simulink model "deadtime_compensation"  (R2020a)
settings: Solver=ode45  StartTime=0.0  StopTime=0.15  FixedStep=0.0000001  RelTol=1e-3
libraries: powerlib_meascontrol x13, powerlib x8, simulink x2, mcbcontrolslib x1
settings Model: Creator=ZJX  LastModifiedBy=ZJX
settings DebuggingCC: UnconnectedInputMsg=none  UnconnectedOutputMsg=none  UnconnectedLineMsg=none
settings ModelReferenceCC: EnableRefExpFcnMdlSchedulingChecks=off
settings RTWCC: Description=Generic Real-Time Target

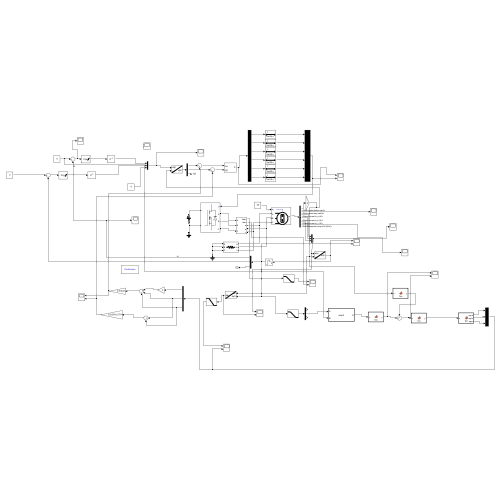
[thumbnail: Simulink's stored preview of the top-level diagram]
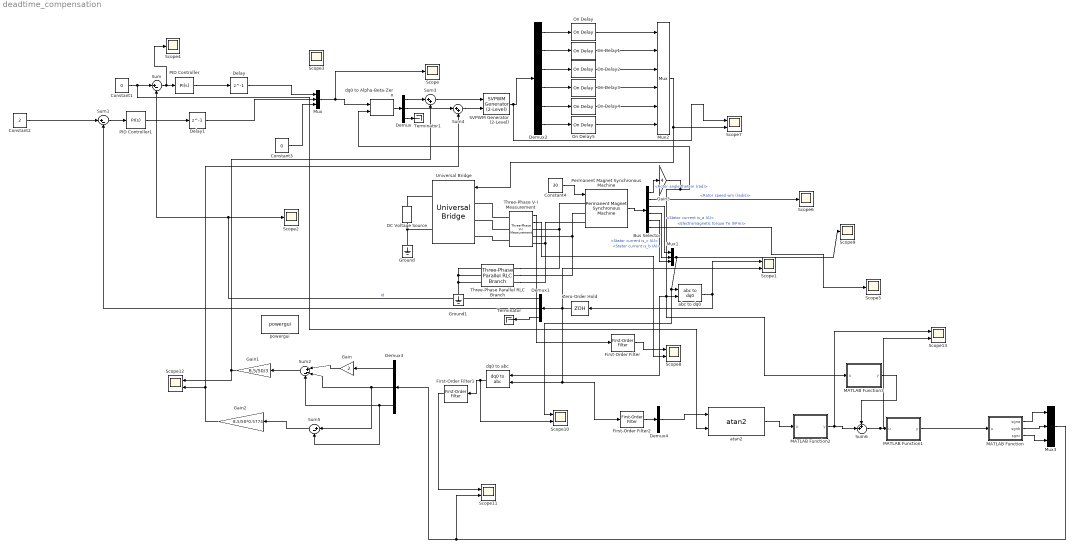
== system deadtime_compensation ==
  Bus Selector : BusSelector  OutputSignals=Rotor angle thetam (rad),Rotor speed wm (rad/s),Stator current is_a (A),Stator current is_b (A),Stator current is_c (A),Electromagnetic torque Te (N*m)
  Constant1 : Constant  Value=0
  Constant2 : Constant  Value=2
  Constant3 : Constant  Value=0
  Constant4 : Constant  Value=30
  DC Voltage Source : powerlib/Electrical Sources/DC Voltage Source  Amplitude=24  Measurements=None
  Delay : Delay  DelayLength=1  InitialCondition=0  SampleTime=0.00005
  Delay1 : Delay  DelayLength=1  InitialCondition=0  SampleTime=0.00005
  Demux{,1,3..4} (4 alike) : Demux  Outputs=3
  Demux2 : Demux  Outputs=6
  First-Order Filter : powerlib_meascontrol/Filters/First-Order Filter  FilterType=Lowpass  Tc=10e-4  Ts=0  Initialize=on  Vac_Init=[0, 0, 60]  Vdc_Init=0  PlotResponse=off  FreqRange="[0,  200,  1]"
  First-Order Filter1 : powerlib_meascontrol/Filters/First-Order Filter  FilterType=Lowpass  Tc=10e-5  Ts=0  Initialize=on  Vac_Init=[0, 0, 60]  Vdc_Init=0  PlotResponse=off  FreqRange="[0,  200,  1]"
  First-Order Filter2 : powerlib_meascontrol/Filters/First-Order Filter  FilterType=Lowpass  Tc=10e-6  Ts=0  Initialize=on  Vac_Init=[0, 0, 60]  Vdc_Init=0  PlotResponse=off  FreqRange="[0,  200,  1]"
  Gain : Gain  Gain=2
  Gain1 : Gain  Gain=8.5/50/3
  Gain2 : Gain  Gain=8.5/50*0.5774
  Gain3 : Gain  Gain=4
  Ground : powerlib/Elements/Ground  LConnTagsString=a
  Ground1 : powerlib/Elements/Ground  LConnTagsString=a
  MATLAB Function : MATLAB Function  TreatAsAtomicUnit=on
  MATLAB Function1 : MATLAB Function  TreatAsAtomicUnit=on
  MATLAB Function2 : MATLAB Function  TreatAsAtomicUnit=on
  MATLAB Function3 : MATLAB Function  TreatAsAtomicUnit=on
  Mux : Mux  Inputs=3
  Mux1 : Mux  Inputs=3
  Mux2 : Mux  Inputs=6
  Mux3 : Mux  Inputs=3
  On Delay{,1..5} (6 alike) : powerlib_meascontrol/Logic/On Delay  DelayType=On delay  delay=0.000005  ic=0  Ts=0
  PID Controller : simulink/Continuous/PID Controller  Controller=PI  Form=Parallel  TimeDomain=Continuous-time  UseExternalTs=off  SampleTime=-1  IntegratorMethod=Forward Euler  ControllerParametersSource=internal  P=0.00017*200  I=0.00017*200* 0.1 / 0.00017  D=0  N=100  UseFilter=on  TunerSelectOption=Frequency Response Based  ZeroCross=off  InitialConditionSource=internal  InitialConditionForIntegrator=0  InitialConditionForFilter=0  DifferentiatorICPrevScaledInput=0  ExternalReset=none  TrackingMode=off  Kt=1  LimitOutput=on  UpperSaturationLimit=1  LowerSaturationLimit=-1  LinearizeAsGain=off  AntiWindupMode=clamping  Kb=1  POutMin=[]  POutMax=[]  IOutMin=[]  IOutMax=[]  DOutMin=[]  DOutMax=[]  NOutMin=[]  NOutMax=[]  SumOutMin=[]  SumOutMax=[]  SaturationOutMin=[]  SaturationOutMax=[]  PParamMin=[]  PParamMax=[]  IParamMin=[]  IParamMax=[]  DParamMin=[]  DParamMax=[]  NParamMin=[]  NParamMax=[]  KbParamMin=[]  KbParamMax=[]  KtParamMin=[]  KtParamMax=[]  KbOutMin=[]  KbOutMax=[]  KtOutMin=[]  KtOutMax=[]  IntegratorOutMin=[]  IntegratorOutMax=[]  FilterOutMin=[]  FilterOutMax=[]  SumI1OutMin=[]  SumI1OutMax=[]  SumI2OutMin=[]  SumI2OutMax=[]  SumI3OutMin=[]  SumI3OutMax=[]  SumI4OutMin=[]  SumI4OutMax=[]  SumDOutMin=[]  SumDOutMax=[]  DifferentiatorOutMin=[]  DifferentiatorOutMax=[]  FilterDiffOutCoefMin=[]  FilterDiffOutCoefMax=[]  ReciprocalOutMin=[]  ReciprocalOutMax=[]  SumDenOutMin=[]  SumDenOutMax=[]  SumNumOutMin=[]  SumNumOutMax=[]  DivideOutMin=[]  DivideOutMax=[]  UdiffTsProdOutMin=[]  UdiffTsProdOutMax=[]  NTsProdOutMin=[]  NTsProdOutMax=[]  UintegralTsProdOutMin=[]  UintegralTsProdOutMax=[]  UngainTsProdOutMin=[]  UngainTsProdOutMax=[]  IntegratorContinuousStateAttributes=''  IntegratorStateMustResolveToSignalObject=off  IntegratorRTWStateStorageClass=Auto  FilterContinuousStateAttributes=''  FilterStateMustResolveToSignalObject=off  FilterRTWStateStorageClass=Auto  ParallelPVariant=InternalParameters  IdealPVariant=Disabled  IVariant=InternalParameters  DVariant=Disabled  IntegratorVariant=Continuous  SatVariant=Enabled  AWVariant=ContClampingParallel  PCopyVariant=Disabled  TRVariant=Disabled  FdbkBlocksVariant=Forward  IdealPFdbkVariant=Disabled  SatFdbkVariant=Disabled  DerivativeFilterVariant=Disabled  NVariant=Disabled  NCopyVariant=Disabled_SignalSpec  FilterICVariant=Disabled  IntegratorICVariant=InternalICs  ExternalResetVariant=Disabled  TRSumVariant=Passthrough  SumFdbkVariant=Disabled  SumVariant=Sum_PI  TsampFilterVariant=InternalTs  TsampNgainVariant=Passthrough  TsampIntegralVariant=Disabled_SignalSpec
  PID Controller1 : simulink/Continuous/PID Controller  Controller=PI  Form=Parallel  TimeDomain=Continuous-time  UseExternalTs=off  SampleTime=-1  IntegratorMethod=Forward Euler  ControllerParametersSource=internal  P=0.00017*200  I=0.00017*200* 0.1 / 0.00017  D=0  N=100  UseFilter=on  TunerSelectOption=Frequency Response Based  ZeroCross=off  InitialConditionSource=internal  InitialConditionForIntegrator=0  InitialConditionForFilter=0  DifferentiatorICPrevScaledInput=0  ExternalReset=none  TrackingMode=off  Kt=1  LimitOutput=on  UpperSaturationLimit=1  LowerSaturationLimit=-1  LinearizeAsGain=off  AntiWindupMode=clamping  Kb=1  POutMin=[]  POutMax=[]  IOutMin=[]  IOutMax=[]  DOutMin=[]  DOutMax=[]  NOutMin=[]  NOutMax=[]  SumOutMin=[]  SumOutMax=[]  SaturationOutMin=[]  SaturationOutMax=[]  PParamMin=[]  PParamMax=[]  IParamMin=[]  IParamMax=[]  DParamMin=[]  DParamMax=[]  NParamMin=[]  NParamMax=[]  KbParamMin=[]  KbParamMax=[]  KtParamMin=[]  KtParamMax=[]  KbOutMin=[]  KbOutMax=[]  KtOutMin=[]  KtOutMax=[]  IntegratorOutMin=[]  IntegratorOutMax=[]  FilterOutMin=[]  FilterOutMax=[]  SumI1OutMin=[]  SumI1OutMax=[]  SumI2OutMin=[]  SumI2OutMax=[]  SumI3OutMin=[]  SumI3OutMax=[]  SumI4OutMin=[]  SumI4OutMax=[]  SumDOutMin=[]  SumDOutMax=[]  DifferentiatorOutMin=[]  DifferentiatorOutMax=[]  FilterDiffOutCoefMin=[]  FilterDiffOutCoefMax=[]  ReciprocalOutMin=[]  ReciprocalOutMax=[]  SumDenOutMin=[]  SumDenOutMax=[]  SumNumOutMin=[]  SumNumOutMax=[]  DivideOutMin=[]  DivideOutMax=[]  UdiffTsProdOutMin=[]  UdiffTsProdOutMax=[]  NTsProdOutMin=[]  NTsProdOutMax=[]  UintegralTsProdOutMin=[]  UintegralTsProdOutMax=[]  UngainTsProdOutMin=[]  UngainTsProdOutMax=[]  IntegratorContinuousStateAttributes=''  IntegratorStateMustResolveToSignalObject=off  IntegratorRTWStateStorageClass=Auto  FilterContinuousStateAttributes=''  FilterStateMustResolveToSignalObject=off  FilterRTWStateStorageClass=Auto  ParallelPVariant=InternalParameters  IdealPVariant=Disabled  IVariant=InternalParameters  DVariant=Disabled  IntegratorVariant=Continuous  SatVariant=Enabled  AWVariant=ContClampingParallel  PCopyVariant=Disabled  TRVariant=Disabled  FdbkBlocksVariant=Forward  IdealPFdbkVariant=Disabled  SatFdbkVariant=Disabled  DerivativeFilterVariant=Disabled  NVariant=Disabled  NCopyVariant=Disabled_SignalSpec  FilterICVariant=Disabled  IntegratorICVariant=InternalICs  ExternalResetVariant=Disabled  TRSumVariant=Passthrough  SumFdbkVariant=Disabled  SumVariant=Sum_PI  TsampFilterVariant=InternalTs  TsampNgainVariant=Passthrough  TsampIntegralVariant=Disabled_SignalSpec
  Permanent Magnet Synchronous Machine : powerlib/Machines/Permanent Magnet Synchronous Machine  NbPhases=3  FluxDistribution=Sinusoidal  RotorType=Round  MechanicalLoad=Speed w  PresetModel=No  ShowDetailedParameters=on  MeasurementBus=off  Resistance=0.1  Inductance=8.5e-3  dqInductances=[8.5e-3,8.5e-3]  La=0.00017  MachineConstant=Torque Constant (N.m / A_peak)  Flux=0.016667  VoltageCst=12.092  TorqueCst=0.1  Flat=120  Mechanical=[0.00027 0.0004924 1 0]  PolePairs=4  InitialConditions=[0,0, 0,0]  InitialConditions5ph=[0 0 0 0 0 0]  RefAngle=Aligned with phase A axis (original Park)  IterativeDiscreteModel=Trapezoidal non iterative  TsBlock=-1  TsPowergui=0
  SVPWM Generator (2-Level) : powerlib_meascontrol/Pulse & Signal Generators/SVPWM Generator (2-Level)  InputType=alpha-beta components  SwitchingPattern=Pattern #1  Fc=20000  ParUref=[0.8 -30 50]  Ts=0
  Scope{,2..6,9} (7 alike) : Scope
  Scope{1,7..8,10..13} (7 alike) : Scope  NumInputPorts=2
  Sum : Sum  Inputs=|+-
  Sum1 : Sum  Inputs=|+-
  Sum2 : Sum  Inputs=|+--
  Sum3 : Sum  Inputs=|++
  Sum4 : Sum  Inputs=|++
  Sum5 : Sum  Inputs=|+-
  Sum6 : Sum  Inputs=++|
  Terminator : Terminator
  Terminator1 : Terminator
  Three-Phase Parallel RLC Branch : powerlib/Elements/Three-Phase Parallel RLC Branch  LConnTagsString=A|B|C  RConnTagsString=A|B|C  BranchType=R  Resistance=2000  Inductance=1e-3  Capacitance=1e-6  Measurements=None
  Three-Phase V-I Measurement : powerlib/Measurements/Three-Phase V-I Measurement  VoltageMeasurement=phase-to-ground  SetLabelV=off  LabelV=Vabc  Vpu=off  VpuLL=off  CurrentMeasurement=yes  SetLabelI=off  LabelI=Iabc  Ipu=off  Pbase=100e6  Vbase=500e3  OutputType=Complex  PhasorSimulation=off  PSBequivalent=0
  Universal Bridge : powerlib/Power Electronics/Universal Bridge  Arms=3  SnubberResistance=1e5  SnubberCapacitance=inf  Device=MOSFET / Diodes  Ron=1e-5  Lon=0  ForwardVoltages="[  0  0  ]"  ForwardVoltage=0  GTOparameters=[ 10e-6 , 20e-6 ]  IGBTparameters=[ 1e-6 , 2e-6 ]  Measurements=None  Measurements_2=None  converterType=Rectifier
  Zero-Order Hold : ZeroOrderHold  SampleTime=0.000025
  abc to dq0 : powerlib_meascontrol/Transformations/abc to dq0  Alignment=Aligned with phase A axis
  atan2 : mcbcontrolslib/atan2  ApproximationMethod=None  NumberOfIterations=11  NumberOfDataPoints=16  InterpMethod=Flat  outputUnit=Radians  TableDataTypeStr=Inherit: Inherit via input
  dq0 to Alpha-Beta-Zero : powerlib_meascontrol/Transformations/dq0 to Alpha-Beta-Zero  Alignment=Aligned with phase A axis
  dq0 to abc : powerlib_meascontrol/Transformations/dq0 to abc  Alignment=Aligned with phase A axis
  powergui : powerlib/powergui  Priority=1  SimulationMode=Continuous  SampleTime=0.000025  frequency=60  Iterations=50  frequencyindice=0  Pbase=100e6  ErrMax=1e-4  UnitsV=kV  UnitsW=MW  buscounter=0  FunctionMessages=off  echomessages=off  EnableUseOfTLC=off  CurrentSourceSwitches=off  DisableSnubberDevices=off  DisableRonSwitches=off  DisableVfSwitches=off  DisplayEquations=off  AutomaticDiscreteSolvers=off  SolverType=Tustin/Backward Euler (TBE)  Interpol=off  ExternalGateDelay=off  methode=off  Ts=100  x0status=blocks  SPID=on  SwTol=0  HookPort=off  NonlinearTolerance=1e-4  nMaxIteration=100  ContinueOnMaxIteration=off  RestoreLinks=warning  ResistiveCurrentMeasurement=off  Frange=[0:2:500]  Ylog=off  Xlog=on  ShowGrid=off  save=off  variable=ZData  structure=0  ZoomFFT=off  StartTime=0.0  cycles=1  DisplayStyle=1  fundamental=60  FreqAxis=off  MaxFrequency=1000  frequencyindicesteady=1  RmsSteady=1  display=off
  wires:
  Constant2/1 -> Sum1/1
  Bus Selector/6 -> Scope5/1  "<Electromagnetic torque Te (N*m)>"
  Demux/3 -> Terminator1/1
  Constant3/1 -> Mux/3
  Sum1/1 -> PID Controller1/1
  Demux1/2 -> Sum1/2
  Bus Selector/2 -> Scope6/1  "<Rotor speed wm (rad/s)>"
  Sum/1 -> Scope4/1, PID Controller/1
  Bus Selector/5 -> Mux1/3  "<Stator current is_c (A)>"
  Constant1/1 -> atan2/2, Sum/1
  Bus Selector/3 -> Mux1/1  "<Stator current is_a (A)>"
  Bus Selector/4 -> Mux1/2  "<Stator current is_b (A)>"
  Mux/1 -> Scope/1, dq0 to Alpha-Beta-Zero/1
  Permanent Magnet Synchronous Machine/1 -> Bus Selector/1
  Demux1/3 -> Terminator/1
  dq0 to Alpha-Beta-Zero/1 -> Demux/1
  Mux1/1 -> Scope10/1, abc to dq0/1, Scope9/1
  Gain3/1 -> MATLAB Function3/1(u), abc to dq0/2, dq0 to abc/2, dq0 to Alpha-Beta-Zero/2
  Demux1/1 -> Sum/2, Scope2/1  "Id"
  Zero-Order Hold/1 -> Scope1/2, dq0 to abc/1, First-Order Filter2/1, Demux1/1
  abc to dq0/1 -> Scope1/1, Zero-Order Hold/1
  Constant4/1 -> Permanent Magnet Synchronous Machine/1
  SVPWM Generator (2-Level)/1 -> Scope7/1, Demux2/1
  Mux2/1 -> Scope7/2, Universal Bridge/1
  Three-Phase V-I Measurement/2 -> Scope8/2
  First-Order Filter/1 -> Scope8/1
  Three-Phase V-I Measurement/1 -> First-Order Filter/1
  Demux2/1 -> On Delay/1
  On Delay/1 -> Mux2/1
  Demux2/2 -> On Delay1/1
  Demux2/3 -> On Delay2/1
  On Delay1/1 -> Mux2/2
  On Delay2/1 -> Mux2/3
  Demux2/4 -> On Delay3/1
  On Delay3/1 -> Mux2/4
  Demux2/5 -> On Delay4/1
  On Delay4/1 -> Mux2/5
  Demux2/6 -> On Delay5/1
  On Delay5/1 -> Mux2/6
  Demux3/1 -> Gain/1
  Gain/1 -> Sum2/1
  Demux3/2 -> Sum5/1, Sum2/2
  Demux3/3 -> Sum5/2, Sum2/3
  Sum2/1 -> Gain1/1
  Demux/1 -> Sum3/1
  Sum3/1 -> SVPWM Generator (2-Level)/1
  Sum4/1 -> SVPWM Generator (2-Level)/2
  Demux/2 -> Sum4/1
  Gain1/1 -> Scope12/1, Sum3/2
  Sum5/1 -> Gain2/1
  Gain2/1 -> Scope12/2, Sum4/2
  dq0 to abc/1 -> Scope10/2, First-Order Filter1/1
  First-Order Filter1/1 -> Scope11/1
  First-Order Filter2/1 -> Demux4/1
  Sum6/1 -> Scope13/2, MATLAB Function1/1(u)
  MATLAB Function1/1(y) -> MATLAB Function/1(u)
  MATLAB Function/1(sgna) -> Mux3/1
  MATLAB Function/2(sgnb) -> Mux3/2
  MATLAB Function/3(sgnc) -> Mux3/3
  Mux3/1 -> Scope11/2, Demux3/1
  MATLAB Function2/1(y) -> Scope13/1, Sum6/2
  atan2/1 -> MATLAB Function2/1(u)
  Bus Selector/1 -> Gain3/1  "<Rotor angle thetam (rad)>"
  MATLAB Function3/1(y) -> Sum6/1
  PID Controller/1 -> Delay/1
  PID Controller1/1 -> Delay1/1
  Demux4/2 -> atan2/1
  Delay/1 -> Mux/1
  Delay1/1 -> Mux/2
  connections:
  Ground/LConn1 -- Universal Bridge/RConn2 -- DC Voltage Source/LConn1
  DC Voltage Source/RConn1 -- Universal Bridge/RConn1
  Three-Phase V-I Measurement/LConn3 -- Universal Bridge/LConn3
  Three-Phase V-I Measurement/LConn2 -- Universal Bridge/LConn2
  Three-Phase V-I Measurement/LConn1 -- Universal Bridge/LConn1
  Three-Phase V-I Measurement/RConn1 -- Three-Phase Parallel RLC Branch/RConn1 -- Permanent Magnet Synchronous Machine/LConn1
  Permanent Magnet Synchronous Machine/LConn2 -- Three-Phase Parallel RLC Branch/RConn2 -- Three-Phase V-I Measurement/RConn2
  Three-Phase V-I Measurement/RConn3 -- Three-Phase Parallel RLC Branch/RConn3 -- Permanent Magnet Synchronous Machine/LConn3
  Three-Phase Parallel RLC Branch/LConn1 -- Ground1/LConn1 -- Three-Phase Parallel RLC Branch/LConn3 -- Three-Phase Parallel RLC Branch/LConn2

== matlab function deadtime_compensation/MATLAB Function ==
  data: u input; sgna output; sgnb output; sgnc output
function [sgna, sgnb, sgnc] = fcn(u)
   
    if 0 < u && u <= pi/6
        sgna = 1;
        sgnb = -1;
        sgnc = -1;
    elseif pi/6 < u && u <= pi/2
        sgna = 1;
        sgnb = 1;
        sgnc = -1;
    elseif pi/2 < u && u <= 5*pi/6
        sgna = -1;
        sgnb = 1;
        sgnc = -1;
    elseif 5*pi/6 < u && u <= 7*pi/6
        sgna = -1;
        sgnb = 1;
        sgnc = 1;
     elseif 7*pi/6 < u && u <= 3*pi/2
        sgna = -1;
        sgnb = -1;
        sgnc = 1;
    elseif 3*pi/2 < u && u <= 11*pi/6
        sgna = 1;
        sgnb = -1;
        sgnc = 1;
    elseif 11*pi/6 < u && u <= 2*pi
        sgna = 1;
        sgnb = -1;
        sgnc = -1;
    else

        sgna = 0;
        sgnb = 0;
        sgnc = 0;
    end
end

== matlab function deadtime_compensation/MATLAB Function2 ==
  data: u input; y output
function y = fcn(u)
    while u > pi/2
        u=  u -pi;
    end

    while u <0
        u = u+pi;
    end

    y =u;
end

== matlab function deadtime_compensation/MATLAB Function3 ==
  data: u input; y output
function y  = fcn(u)

y = mod(u,2*pi);

== matlab function deadtime_compensation/MATLAB Function1 ==
  data: u input; y output
function y = fcn(u)

y = mod(u,2*pi);
